simulink model "VehCtrlMdel240926_2018b_amkspdlimit"  (R2019b)
settings: Solver=FixedStepDiscrete  StartTime=0.0  StopTime=20  FixedStep=0.0005  RelTol=1e-3  EnableMultiTasking=on
values from neighbouring files (symbols this model uses):
  Ax_OffSet = 0.0    [VehCtrlMdelDictionary.sldd]
  Ay_OffSet = 0.0    [VehCtrlMdelDictionary.sldd]
  Caf = 460.0    [VehCtrlMdelDictionary.sldd]
  Car = 440.0    [VehCtrlMdelDictionary.sldd]
  dwf = 1.2    [VehCtrlMdelDictionary.sldd]
  dwr = 1.2    [VehCtrlMdelDictionary.sldd]
  h = 0.29    [VehCtrlMdelDictionary.sldd]
  i1 = 11.42    [VehCtrlMdelDictionary.sldd]
  i2 = 3.727    [VehCtrlMdelDictionary.sldd]
  Iz = 105.0    [VehCtrlMdelDictionary.sldd]
  Kc = 1.0    [VehCtrlMdelDictionary.sldd]
  Ki = 1.0    [VehCtrlMdelDictionary.sldd]
  Kp = 2.0    [VehCtrlMdelDictionary.sldd]
  Ldwf = 1.2    [VehCtrlMdelDictionary.sldd]
  Ldwr = 1.16    [VehCtrlMdelDictionary.sldd]
  lf = 0.761    [VehCtrlMdelDictionary.sldd]
  lr = 0.831    [VehCtrlMdelDictionary.sldd]
  m = 340.0    [VehCtrlMdelDictionary.sldd]
  Offset_Angle = 0.0    [VehCtrlMdelDictionary.sldd]
  Qa = 0.1    [VehCtrlMdelDictionary.sldd]
  Ra = 2.0    [VehCtrlMdelDictionary.sldd]
  Rt = 0.2    [VehCtrlMdelDictionary.sldd]
  thr1 = 2.0    [VehCtrlMdelDictionary.sldd]
  thr2 = 0.5    [VehCtrlMdelDictionary.sldd]
  thr3 = 0.8    [VehCtrlMdelDictionary.sldd]
  thr4 = 0.5    [VehCtrlMdelDictionary.sldd]
  thr5 = -0.5    [VehCtrlMdelDictionary.sldd]
  TrqRquRate = 0.1    [VehCtrlMdelDictionary.sldd]
  YawRate_OffSet = 0.0    [VehCtrlMdelDictionary.sldd]
undefined symbols (not defined in the file or in its folder): DiscIntNeverNeededParam, I_AN06_5V, I_AN07_5V, I_AN08_5V, I_AN09_5V, I_SW01_L, I_SW03_L, I_SW04_L, O_SW01_LS0A4, O_SW12_HS1A, O_SW13_HS1A, O_SW14_HS1A, O_SW15_HS1A, PWM3
libraries: simulink x152, ec5744lib x129, canmsglib x18
(part 5 of 6)

== system VehCtrlMdel240926_2018b_amkspdlimit/Input_Processing/Subsystem/WhlSlpageJudgment/速差判断 ==
  note: 输出“1”代表判定有效
  <VxFL_mps> : Inport
  <VxFR_mps> : Inport  Port=2
  <VxRL_mps> : Inport  Port=3
  <VxRR_mps> : Inport  Port=4
  VehSpd_mps : Inport  Port=5
  In6 : Inport  Port=6
  AND{,1..3} (4 alike) : Logic  AllPortsSameDT=off  OutDataTypeStr=boolean
  Abs{,1..3} (4 alike) : Abs
  Add{,1..3} (4 alike) : Sum  Inputs=+-
  Bus Selector1 : BusSelector  OutputSignals=WhlSpdii_mps.WhlSpdRL_Valid,WhlSpdii_mps.WhlSpdRR_Valid,WhlSpdii_mps.WhlSpdFR_Valid,WhlSpdii_mps.WhlSpdFL_Valid
  Compare To Constant{,1..3} (4 alike) : simulink/Logic and Bit Operations/Compare To Constant  relop=<=  const=thr1  OutDataTypeStr=boolean
  y : Outport
  y1 : Outport  Port=2
  y2 : Outport  Port=3
  y3 : Outport  Port=4
  wires:
  Add2/1 -> Abs2/1
  Abs1/1 -> Compare To Constant1/1
  <VxRR_mps>/1 -> Add3/1
  Add3/1 -> Abs3/1
  Add/1 -> Abs/1
  [VehSpd_mps] -> Add1/2
  <VxRL_mps>/1 -> Add2/1
  <VxFR_mps>/1 -> Add1/1
  Compare To Constant1/1 -> AND2/1
  Compare To Constant3/1 -> AND1/1
  Abs3/1 -> Compare To Constant3/1
  [VehSpd_mps] -> Add/2
  [VehSpd_mps] -> Add2/2
  [VehSpd_mps] -> Add3/2
  Abs/1 -> Compare To Constant/1
  Add1/1 -> Abs1/1
  Abs2/1 -> Compare To Constant2/1
  <VxFL_mps>/1 -> Add/1
  Compare To Constant2/1 -> AND/1
  Compare To Constant/1 -> AND3/1
  VehSpd_mps/1 -> [VehSpd_mps]
  In6/1 -> Bus Selector1/1
  Bus Selector1/1 -> AND/2  "<WhlSpdRL_Valid>"
  Bus Selector1/2 -> AND1/2  "<WhlSpdRR_Valid>"
  Bus Selector1/3 -> AND2/2  "<WhlSpdFR_Valid>"
  Bus Selector1/4 -> AND3/2  "<WhlSpdFL_Valid>"
  AND3/1 -> y/1
  AND2/1 -> y1/1
  AND1/1 -> y3/1
  AND/1 -> y2/1

== system VehCtrlMdel240926_2018b_amkspdlimit/Input_Processing/Subsystem/WhlSpdSelect/Filter ==
  In : Inport
  Add : Sum
  Constant : Constant  Value=single(0)
  Constant1 : Constant  Value=single(100)
  Constant2 : Constant  Value=single(15)
  Constant3 : Constant  Value=single(-15)
  Gain : Gain  Gain=0
  Gain1 : Gain
  Rate Limiter Dynamic : simulink/Discontinuities/Rate Limiter Dynamic
      settings: SourceProductName=Simulink
  Saturation Dynamic : simulink/Discontinuities/Saturation Dynamic  OutMin=[]  OutMax=[]  OutDataTypeStr=Inherit: Same as second input  OutDataType=fixdt(1, 16)  OutScaling=2^-10  DoSatur=off
  Unit Delay : UnitDelay  SampleTime=-1  HasFrameUpgradeWarning=on
  VehVxEst_mps : Outport
  wires:
  In/1 -> Saturation Dynamic/2
  Saturation Dynamic/1 -> Rate Limiter Dynamic/2
  Constant1/1 -> Saturation Dynamic/1
  Constant/1 -> Saturation Dynamic/3
  Unit Delay/1 -> Gain/1
  Gain/1 -> Add/1
  Gain1/1 -> Add/2
  Rate Limiter Dynamic/1 -> Gain1/1, Unit Delay/1
  Add/1 -> VehVxEst_mps/1
  Constant2/1 -> Rate Limiter Dynamic/1
  Constant3/1 -> Rate Limiter Dynamic/3

== system VehCtrlMdel240926_2018b_amkspdlimit/Input_Processing/Subsystem/WhlSpdSelect/Subsystem ==
  <VxFL_mps> : Inport
  <VxFR_mps> : Inport  Port=2
  <VxRL_mps> : Inport  Port=3
  <VxRR_mps> : Inport  Port=4
  Add3 : Sum  Inputs=++++
  Add4 : Sum  Inputs=+--
  Gain1 : Gain  Gain=1/2
  Min3 : MinMax  Function=max  Inputs=4
  Min4 : MinMax  Inputs=4
  Subsystem : Subsystem  Commented=on
  MiddleWhlSpd_mps : Outport
  wires:
  Add4/1 -> Gain1/1
  Add3/1 -> Add4/1
  Min3/1 -> Add4/3
  <VxRR_mps>/1 -> Min3/4, Add3/1, Min4/4
  <VxRL_mps>/1 -> Min3/3, Min4/3, Add3/2
  <VxFR_mps>/1 -> Min4/2, Min3/2, Add3/3
  Min4/1 -> Add4/2
  <VxFL_mps>/1 -> Add3/4, Min4/1, Min3/1
  Gain1/1 -> MiddleWhlSpd_mps/1  "MaxWhlSpd_mps"

== system VehCtrlMdel240926_2018b_amkspdlimit/Input/AMKMCU_Receive/FLAMKMCU/AMKMCU_state/MCU_state ==
  ID : Inport
  Msg : Inport  Port=2
  Enable : EnablePort
  Bus Creator : BusCreator  Inputs=12
  CAN Unpack : canmsglib/CAN Unpack  CANdbFile=d:\Users\YJR\Desktop\低压组\amk电机\DRe20_dbc_v1.16\DRe20_dbc_v1.16_CAN2.dbc  MsgList=MCFL_ActualValue1  MsgName=MCFL_ActualValue1  MsgIDType=Standard (11-bit identifier)  MsgIdentifier=640  MsgLength=8  SignalInfo={'MCFL_ActualTorque','32','16','LE','signed','Standard','0','0.0098','0','-Inf','Inf';'MCFL_ActualVelocity','48','16','LE','signed','Standard','0','1','0','-Inf','Inf';'MCFL_DCVoltage','16','16','LE','unsigned','Standard','0','1','0','-Inf','Inf';'MCFL_bDCOn','12','1','LE','unsigned','Standard','0','1','0','0','1';'MCFL_bDerating','15','1','LE','unsigned','Standard','0','1','0','0','1';'MCFL_bError','9','1','LE','unsigned','Standard','0','1','0','0','1';'MCFL_bInverterOn','14','1','LE','unsigned','Standard','0','1','0','0','1';'MCFL_bQuitDCOn','11','1','LE','unsigned','Standard','0','1','0','0','1';'MCFL_bQuitInverterOn','13','1','LE','unsigned','Standard','0','1','0','0','1';'MCFL_bReserve','0','8','LE','unsigned','Standard','0','1','0','0','255';'MCFL_bSystemReady','8','1','LE','unsigned','Standard','0','1','0','0','1';'MCFL_bWarn','10','1','LE','unsigned','Standard','0','1','0','0','1'}  IDPort=off  TimestampPort=off  ErrorPort=off  RemotePort=off  LengthPort=off  StatusPort=off  ApplyMinMax=off
      settings: SourceProductName=Simulink Real-Time  SourceProductBaseCode=XP  DataFormat=CANdb specified signals
  CANUnPackMessage4 : ec5744lib/RapidECU_U3/04CANCommunication/CANUnPackMessage  datalength=8  canmessagetype=Standard(11-bit ID)  sampletime=-1
      settings: SourceProductName=ECUCoder for MPC5744
  Gain : Gain  Gain=-1
  MeaModule1 : ec5744lib/RapidECU_U3/07Calibration/MeaModule  signal=MCFL_ActualVelocity
      settings: SourceProductName=ECUCoder for MPC5744
  MeaModule2 : ec5744lib/RapidECU_U3/07Calibration/MeaModule  signal=MCFL_DCVoltage
      settings: SourceProductName=ECUCoder for MPC5744
  MeaModule3 : ec5744lib/RapidECU_U3/07Calibration/MeaModule  signal=MCFL_bDCOn
      settings: SourceProductName=ECUCoder for MPC5744
  MeaModule4 : ec5744lib/RapidECU_U3/07Calibration/MeaModule  signal=MCFL_bError
      settings: SourceProductName=ECUCoder for MPC5744
  MeaModule5 : ec5744lib/RapidECU_U3/07Calibration/MeaModule  signal=MCFL_bInverterOn
      settings: SourceProductName=ECUCoder for MPC5744
  MeaModule6 : ec5744lib/RapidECU_U3/07Calibration/MeaModule  signal=MCFL_bQuitDCOn
      settings: SourceProductName=ECUCoder for MPC5744
  MeaModule7 : ec5744lib/RapidECU_U3/07Calibration/MeaModule  signal=MCFL_bQuitInverterOn
      settings: SourceProductName=ECUCoder for MPC5744
  MeaModule8 : ec5744lib/RapidECU_U3/07Calibration/MeaModule  signal=MCFL_bSystemReady
      settings: SourceProductName=ECUCoder for MPC5744
  MeaModule9 : ec5744lib/RapidECU_U3/07Calibration/MeaModule  signal=MCFL_ActualTorque
      settings: SourceProductName=ECUCoder for MPC5744
  FLAMKMCUtoVCU1 : Outport  VectorParamsAs1DForOutWhenUnconnected=off
  wires:
  Msg/1 -> CANUnPackMessage4/2
  ID/1 -> CANUnPackMessage4/1
  CANUnPackMessage4/1 -> CAN Unpack/1
  CAN Unpack/1 -> MeaModule9/1  "MCFL_ActualTorque"
  CAN Unpack/2 -> Gain/1  "MCFL_ActualVelocity"
  CAN Unpack/3 -> MeaModule2/1  "MCFL_DCVoltage"
  CAN Unpack/4 -> MeaModule3/1  "MCFL_bDCOn"
  CAN Unpack/5 -> Bus Creator/5  "MCFL_bDerating"
  CAN Unpack/6 -> MeaModule4/1  "MCFL_bError"
  CAN Unpack/7 -> MeaModule5/1  "MCFL_bInverterOn"
  CAN Unpack/8 -> MeaModule6/1  "MCFL_bQuitDCOn"
  CAN Unpack/9 -> MeaModule7/1  "MCFL_bQuitInverterOn"
  CAN Unpack/10 -> Bus Creator/10  "MCFL_bReserve"
  CAN Unpack/11 -> MeaModule8/1  "MCFL_bSystemReady"
  CAN Unpack/12 -> Bus Creator/12  "MCFL_bWarn"
  Bus Creator/1 -> FLAMKMCUtoVCU1/1  "FLAMKMCUtoVCU1"
  MeaModule1/1 -> Bus Creator/2
  MeaModule2/1 -> Bus Creator/3
  MeaModule3/1 -> Bus Creator/4
  MeaModule4/1 -> Bus Creator/6
  MeaModule5/1 -> Bus Creator/7
  MeaModule6/1 -> Bus Creator/8
  MeaModule7/1 -> Bus Creator/9
  MeaModule8/1 -> Bus Creator/11
  Gain/1 -> MeaModule1/1
  MeaModule9/1 -> Bus Creator/1  "MCFL_ActualTorque"

== system VehCtrlMdel240926_2018b_amkspdlimit/Input/AMKMCU_Receive/FLAMKMCU/AMKMCU_state1/MCU_state ==
  ID : Inport
  Msg : Inport  Port=2
  Enable : EnablePort
  CAN Unpack : canmsglib/CAN Unpack  CANdbFile=d:\Users\YJR\Desktop\低压组\amk电机\DRe20_dbc_v1.16\DRe20_dbc_v1.16_CAN2.dbc  MsgList=MCFL_ActualValue2  MsgName=MCFL_ActualValue2  MsgIDType=Standard (11-bit identifier)  MsgIdentifier=642  MsgLength=8  SignalInfo={'MCFL_DiagnosticNum','0','32','LE','unsigned','Standard','0','1','0','-Inf','Inf';'MCFL_ErrorInfo','32','32','LE','unsigned','Standard','0','1','0','-Inf','Inf'}  IDPort=off  TimestampPort=off  ErrorPort=off  RemotePort=off  LengthPort=off  StatusPort=off  ApplyMinMax=off
      settings: SourceProductName=Simulink Real-Time  SourceProductBaseCode=XP  DataFormat=CANdb specified signals
  CANUnPackMessage4 : ec5744lib/RapidECU_U3/04CANCommunication/CANUnPackMessage  datalength=8  canmessagetype=Standard(11-bit ID)  sampletime=-1
      settings: SourceProductName=ECUCoder for MPC5744
  MeaModule1 : ec5744lib/RapidECU_U3/07Calibration/MeaModule  signal=MCFL_ErrorInfo
      settings: SourceProductName=ECUCoder for MPC5744
  MCFL_DiagnosticNum : Outport  VectorParamsAs1DForOutWhenUnconnected=off
  MCFL_ErrorInfo : Outport  Port=2  VectorParamsAs1DForOutWhenUnconnected=off
  wires:
  CANUnPackMessage4/1 -> CAN Unpack/1
  ID/1 -> CANUnPackMessage4/1
  Msg/1 -> CANUnPackMessage4/2
  CAN Unpack/1 -> MCFL_DiagnosticNum/1  "MCFL_DiagnosticNum"
  CAN Unpack/2 -> MeaModule1/1  "MCFL_ErrorInfo"
  MeaModule1/1 -> MCFL_ErrorInfo/1

== system VehCtrlMdel240926_2018b_amkspdlimit/Input/AMKMCU_Receive/FLAMKMCU/AMKMCU_state2/MCU_state ==
  ID : Inport
  Msg : Inport  Port=2
  Enable : EnablePort
  CAN Unpack : canmsglib/CAN Unpack  CANdbFile=d:\Users\YJR\Desktop\低压组\amk电机\DRe20_dbc_v1.16\DRe20_dbc_v1.16_CAN2.dbc  MsgList=MCFL_ActualValue3  MsgName=MCFL_ActualValue3  MsgIDType=Standard (11-bit identifier)  MsgIdentifier=644  MsgLength=6  SignalInfo={'MCFL_TempIGBT','32','16','LE','unsigned','Standard','0','0.1','0','-Inf','Inf';'MCFL_TempInverter','16','16','LE','unsigned','Standard','0','0.1','0','-Inf','Inf';'MCFL_TempMotor','0','16','LE','unsigned','Standard','0','0.1','0','-Inf','Inf'}  IDPort=off  TimestampPort=off  ErrorPort=off  RemotePort=off  LengthPort=off  StatusPort=off  ApplyMinMax=off
      settings: SourceProductName=Simulink Real-Time  SourceProductBaseCode=XP  DataFormat=CANdb specified signals
  CANUnPackMessage4 : ec5744lib/RapidECU_U3/04CANCommunication/CANUnPackMessage  datalength=6  canmessagetype=Standard(11-bit ID)  sampletime=-1
      settings: SourceProductName=ECUCoder for MPC5744
  MeaModule1 : ec5744lib/RapidECU_U3/07Calibration/MeaModule  signal=MCFL_TempIGBT
      settings: SourceProductName=ECUCoder for MPC5744
  MeaModule2 : ec5744lib/RapidECU_U3/07Calibration/MeaModule  signal=MCFL_TempInverter
      settings: SourceProductName=ECUCoder for MPC5744
  MeaModule3 : ec5744lib/RapidECU_U3/07Calibration/MeaModule  signal=MCFL_TempMotor
      settings: SourceProductName=ECUCoder for MPC5744
  MCFL_TempIGBT : Outport  VectorParamsAs1DForOutWhenUnconnected=off
  MCFL_TempInverter : Outport  Port=2  VectorParamsAs1DForOutWhenUnconnected=off
  MCFL_TempMotor : Outport  Port=3  VectorParamsAs1DForOutWhenUnconnected=off
  wires:
  Msg/1 -> CANUnPackMessage4/2
  ID/1 -> CANUnPackMessage4/1
  CANUnPackMessage4/1 -> CAN Unpack/1
  CAN Unpack/1 -> MeaModule1/1  "MCFL_TempIGBT"
  CAN Unpack/2 -> MeaModule2/1  "MCFL_TempInverter"
  CAN Unpack/3 -> MeaModule3/1  "MCFL_TempMotor"
  MeaModule1/1 -> MCFL_TempIGBT/1
  MeaModule2/1 -> MCFL_TempInverter/1
  MeaModule3/1 -> MCFL_TempMotor/1

== system VehCtrlMdel240926_2018b_amkspdlimit/Input/AMKMCU_Receive/FRAMKMCU/AMKMCU_state/MCU_state ==
  ID : Inport
  Msg : Inport  Port=2
  Enable : EnablePort
  CAN Unpack : canmsglib/CAN Unpack  CANdbFile=d:\Users\YJR\Desktop\低压组\amk电机\DRe20_dbc_v1.16\DRe20_dbc_v1.16_CAN2.dbc  MsgList=MCFR_ActualValue1  MsgName=MCFR_ActualValue1  MsgIDType=Standard (11-bit identifier)  MsgIdentifier=641  MsgLength=8  SignalInfo={'MCFR_ActualTorque','32','16','LE','signed','Standard','0','0.0098','0','-Inf','Inf';'MCFR_ActualVelocity','48','16','LE','signed','Standard','0','1','0','-Inf','Inf';'MCFR_DCVoltage','16','16','LE','unsigned','Standard','0','1','0','-Inf','Inf';'MCFR_bDCOn','12','1','LE','unsigned','Standard','0','1','0','0','1';'MCFR_bDerating','15','1','LE','unsigned','Standard','0','1','0','0','1';'MCFR_bError','9','1','LE','unsigned','Standard','0','1','0','0','1';'MCFR_bInverterOn','14','1','LE','unsigned','Standard','0','1','0','0','1';'MCFR_bQuitDCOn','11','1','LE','unsigned','Standard','0','1','0','0','1';'MCFR_bQuitInverterOn','13','1','LE','unsigned','Standard','0','1','0','0','1';'MCFR_bReserve','0','8','LE','unsigned','Standard','0','1','0','0','255';'MCFR_bSystemReady','8','1','LE','unsigned','Standard','0','1','0','0','1';'MCFR_bWarn','10','1','LE','unsigned','Standard','0','1','0','0','1'}  IDPort=off  TimestampPort=off  ErrorPort=off  RemotePort=off  LengthPort=off  StatusPort=off  ApplyMinMax=off
      settings: SourceProductName=Simulink Real-Time  SourceProductBaseCode=XP  DataFormat=CANdb specified signals
  CANUnPackMessage4 : ec5744lib/RapidECU_U3/04CANCommunication/CANUnPackMessage  datalength=8  canmessagetype=Standard(11-bit ID)  sampletime=-1
      settings: SourceProductName=ECUCoder for MPC5744
  MeaModule1 : ec5744lib/RapidECU_U3/07Calibration/MeaModule  signal=MCFR_ActualVelocity
      settings: SourceProductName=ECUCoder for MPC5744
  MeaModule2 : ec5744lib/RapidECU_U3/07Calibration/MeaModule  signal=MCFR_DCVoltage
      settings: SourceProductName=ECUCoder for MPC5744
  MeaModule3 : ec5744lib/RapidECU_U3/07Calibration/MeaModule  signal=MCFR_bDCOn
      settings: SourceProductName=ECUCoder for MPC5744
  MeaModule4 : ec5744lib/RapidECU_U3/07Calibration/MeaModule  signal=MCFR_bError
      settings: SourceProductName=ECUCoder for MPC5744
  MeaModule5 : ec5744lib/RapidECU_U3/07Calibration/MeaModule  signal=MCFR_bInverterOn
      settings: SourceProductName=ECUCoder for MPC5744
  MeaModule6 : ec5744lib/RapidECU_U3/07Calibration/MeaModule  signal=MCFR_bQuitInverterOn
      settings: SourceProductName=ECUCoder for MPC5744
  MeaModule7 : ec5744lib/RapidECU_U3/07Calibration/MeaModule  signal=MCFR_bSystemReady
      settings: SourceProductName=ECUCoder for MPC5744
  MeaModule8 : ec5744lib/RapidECU_U3/07Calibration/MeaModule  signal=MCFR_ActualTorque
      settings: SourceProductName=ECUCoder for MPC5744
  MCFR_ActualTorque : Outport  VectorParamsAs1DForOutWhenUnconnected=off
  MCFR_ActualVelocity : Outport  Port=2  VectorParamsAs1DForOutWhenUnconnected=off
  MCFR_DCVoltage : Outport  Port=3  VectorParamsAs1DForOutWhenUnconnected=off
  MCFR_bDCOn : Outport  Port=4  VectorParamsAs1DForOutWhenUnconnected=off
  MCFR_bDerating : Outport  Port=5  VectorParamsAs1DForOutWhenUnconnected=off
  MCFR_bError : Outport  Port=6  VectorParamsAs1DForOutWhenUnconnected=off
  MCFR_bInverterOn : Outport  Port=7  VectorParamsAs1DForOutWhenUnconnected=off
  MCFR_bQuitDCOn : Outport  Port=8  VectorParamsAs1DForOutWhenUnconnected=off
  MCFR_bQuitInverterOn : Outport  Port=9  VectorParamsAs1DForOutWhenUnconnected=off
  MCFR_bReserve : Outport  Port=10  VectorParamsAs1DForOutWhenUnconnected=off
  MCFR_bSystemReady : Outport  Port=11  VectorParamsAs1DForOutWhenUnconnected=off
  MCFR_bWarn : Outport  Port=12  VectorParamsAs1DForOutWhenUnconnected=off
  wires:
  CANUnPackMessage4/1 -> CAN Unpack/1
  ID/1 -> CANUnPackMessage4/1
  Msg/1 -> CANUnPackMessage4/2
  CAN Unpack/1 -> MeaModule8/1  "MCFR_ActualTorque"
  CAN Unpack/2 -> MeaModule1/1  "MCFR_ActualVelocity"
  CAN Unpack/4 -> MeaModule3/1  "MCFR_bDCOn"
  CAN Unpack/3 -> MeaModule2/1  "MCFR_DCVoltage"
  CAN Unpack/7 -> MeaModule5/1  "MCFR_bInverterOn"
  CAN Unpack/5 -> MCFR_bDerating/1  "MCFR_bDerating"
  CAN Unpack/6 -> MeaModule4/1  "MCFR_bError"
  CAN Unpack/8 -> MCFR_bQuitDCOn/1  "MCFR_bQuitDCOn"
  CAN Unpack/9 -> MeaModule6/1  "MCFR_bQuitInverterOn"
  CAN Unpack/10 -> MCFR_bReserve/1  "MCFR_bReserve"
  CAN Unpack/11 -> MeaModule7/1  "MCFR_bSystemReady"
  CAN Unpack/12 -> MCFR_bWarn/1  "MCFR_bWarn"
  MeaModule1/1 -> MCFR_ActualVelocity/1
  MeaModule2/1 -> MCFR_DCVoltage/1
  MeaModule3/1 -> MCFR_bDCOn/1
  MeaModule4/1 -> MCFR_bError/1
  MeaModule5/1 -> MCFR_bInverterOn/1
  MeaModule6/1 -> MCFR_bQuitInverterOn/1
  MeaModule7/1 -> MCFR_bSystemReady/1
  MeaModule8/1 -> MCFR_ActualTorque/1  "MCFR_ActualTorque"

== system VehCtrlMdel240926_2018b_amkspdlimit/Input/AMKMCU_Receive/FRAMKMCU/AMKMCU_state1/MCU_state ==
  ID : Inport
  Msg : Inport  Port=2
  Enable : EnablePort
  CAN Unpack : canmsglib/CAN Unpack  CANdbFile=d:\Users\YJR\Desktop\低压组\amk电机\DRe20_dbc_v1.16\DRe20_dbc_v1.16_CAN2.dbc  MsgList=MCFR_ActualValue2  MsgName=MCFR_ActualValue2  MsgIDType=Standard (11-bit identifier)  MsgIdentifier=643  MsgLength=8  SignalInfo={'MCFR_DiagnosticNum','0','32','LE','unsigned','Standard','0','1','0','-Inf','Inf';'MCFR_ErrorInfo','32','32','LE','unsigned','Standard','0','1','0','-Inf','Inf'}  IDPort=off  TimestampPort=off  ErrorPort=off  RemotePort=off  LengthPort=off  StatusPort=off  ApplyMinMax=off
      settings: SourceProductName=Simulink Real-Time  SourceProductBaseCode=XP  DataFormat=CANdb specified signals
  CANUnPackMessage4 : ec5744lib/RapidECU_U3/04CANCommunication/CANUnPackMessage  datalength=8  canmessagetype=Standard(11-bit ID)  sampletime=-1
      settings: SourceProductName=ECUCoder for MPC5744
  MeaModule1 : ec5744lib/RapidECU_U3/07Calibration/MeaModule  signal=MCFR_ErrorInfo
      settings: SourceProductName=ECUCoder for MPC5744
  MCFR_DiagnosticNum : Outport  VectorParamsAs1DForOutWhenUnconnected=off
  MCFR_ErrorInfo : Outport  Port=2  VectorParamsAs1DForOutWhenUnconnected=off
  wires:
  Msg/1 -> CANUnPackMessage4/2
  ID/1 -> CANUnPackMessage4/1
  CANUnPackMessage4/1 -> CAN Unpack/1
  CAN Unpack/1 -> MCFR_DiagnosticNum/1  "MCFR_DiagnosticNum"
  CAN Unpack/2 -> MeaModule1/1  "MCFR_ErrorInfo"
  MeaModule1/1 -> MCFR_ErrorInfo/1

== system VehCtrlMdel240926_2018b_amkspdlimit/Input/AMKMCU_Receive/FRAMKMCU/AMKMCU_state2/MCU_state ==
  ID : Inport
  Msg : Inport  Port=2
  Enable : EnablePort
  CAN Unpack : canmsglib/CAN Unpack  CANdbFile=d:\Users\YJR\Desktop\低压组\amk电机\DRe20_dbc_v1.16\DRe20_dbc_v1.16_CAN2.dbc  MsgList=MCFR_ActualValue3  MsgName=MCFR_ActualValue3  MsgIDType=Standard (11-bit identifier)  MsgIdentifier=645  MsgLength=6  SignalInfo={'MCFR_TempIGBT','32','16','LE','unsigned','Standard','0','0.1','0','-Inf','Inf';'MCFR_TempInverter','16','16','LE','unsigned','Standard','0','0.1','0','-Inf','Inf';'MCFR_TempMotor','0','16','LE','unsigned','Standard','0','0.1','0','-Inf','Inf'}  IDPort=off  TimestampPort=off  ErrorPort=off  RemotePort=off  LengthPort=off  StatusPort=off  ApplyMinMax=off
      settings: SourceProductName=Simulink Real-Time  SourceProductBaseCode=XP  DataFormat=CANdb specified signals
  CANUnPackMessage4 : ec5744lib/RapidECU_U3/04CANCommunication/CANUnPackMessage  datalength=6  canmessagetype=Standard(11-bit ID)  sampletime=-1
      settings: SourceProductName=ECUCoder for MPC5744
  MeaModule1 : ec5744lib/RapidECU_U3/07Calibration/MeaModule  signal=MCFR_TempIGBT
      settings: SourceProductName=ECUCoder for MPC5744
  MeaModule2 : ec5744lib/RapidECU_U3/07Calibration/MeaModule  signal=MCFR_TempInverter
      settings: SourceProductName=ECUCoder for MPC5744
  MeaModule3 : ec5744lib/RapidECU_U3/07Calibration/MeaModule  signal=MCFR_TempMotor
      settings: SourceProductName=ECUCoder for MPC5744
  MCFR_TempIGBT : Outport  VectorParamsAs1DForOutWhenUnconnected=off
  MCFR_TempInverter : Outport  Port=2  VectorParamsAs1DForOutWhenUnconnected=off
  MCFR_TempMotor : Outport  Port=3  VectorParamsAs1DForOutWhenUnconnected=off
  wires:
  CANUnPackMessage4/1 -> CAN Unpack/1
  ID/1 -> CANUnPackMessage4/1
  Msg/1 -> CANUnPackMessage4/2
  CAN Unpack/1 -> MeaModule1/1  "MCFR_TempIGBT"
  CAN Unpack/2 -> MeaModule2/1  "MCFR_TempInverter"
  CAN Unpack/3 -> MeaModule3/1  "MCFR_TempMotor"
  MeaModule1/1 -> MCFR_TempIGBT/1
  MeaModule2/1 -> MCFR_TempInverter/1
  MeaModule3/1 -> MCFR_TempMotor/1

== system VehCtrlMdel240926_2018b_amkspdlimit/Input_Processing/Subsystem/WhlSlpageJudgment/加速度差判断/Filter ==
  In : Inport
  Add : Sum
  Constant : Constant  Value=single(-100)
  Constant1 : Constant  Value=single(100)
  Constant2 : Constant  Value=single(100)
  Constant3 : Constant  Value=single(-100)
  Gain : Gain  Gain=0.3
  Gain1 : Gain  Gain=0.7
  Rate Limiter Dynamic : simulink/Discontinuities/Rate Limiter Dynamic
      settings: SourceProductName=Simulink
  Saturation Dynamic : simulink/Discontinuities/Saturation Dynamic  OutMin=[]  OutMax=[]  OutDataTypeStr=Inherit: Same as second input  OutDataType=fixdt(1, 16)  OutScaling=2^-10  DoSatur=off
  Unit Delay : UnitDelay  SampleTime=-1  HasFrameUpgradeWarning=on
  Out : Outport
  wires:
  In/1 -> Saturation Dynamic/2
  Saturation Dynamic/1 -> Rate Limiter Dynamic/2
  Constant1/1 -> Saturation Dynamic/1
  Constant/1 -> Saturation Dynamic/3
  Constant2/1 -> Rate Limiter Dynamic/1
  Constant3/1 -> Rate Limiter Dynamic/3
  Unit Delay/1 -> Gain/1
  Gain/1 -> Add/1
  Add/1 -> Out/1
  Gain1/1 -> Add/2
  Rate Limiter Dynamic/1 -> Gain1/1, Unit Delay/1

== system VehCtrlMdel240926_2018b_amkspdlimit/Input_Processing/Subsystem/WhlSlpageJudgment/加速度差判断/Filter1 ==
  In : Inport
  Add : Sum
  Constant : Constant  Value=single(-100)
  Constant1 : Constant  Value=single(100)
  Constant2 : Constant  Value=single(100)
  Constant3 : Constant  Value=single(-100)
  Gain : Gain  Gain=0.3
  Gain1 : Gain  Gain=0.7
  Rate Limiter Dynamic : simulink/Discontinuities/Rate Limiter Dynamic
      settings: SourceProductName=Simulink
  Saturation Dynamic : simulink/Discontinuities/Saturation Dynamic  OutMin=[]  OutMax=[]  OutDataTypeStr=Inherit: Same as second input  OutDataType=fixdt(1, 16)  OutScaling=2^-10  DoSatur=off
  Unit Delay : UnitDelay  SampleTime=-1  HasFrameUpgradeWarning=on
  Out : Outport
  wires:
  Rate Limiter Dynamic/1 -> Unit Delay/1, Gain1/1
  Gain1/1 -> Add/2
  Add/1 -> Out/1
  Gain/1 -> Add/1
  Unit Delay/1 -> Gain/1
  Constant3/1 -> Rate Limiter Dynamic/3
  Constant2/1 -> Rate Limiter Dynamic/1
  Constant/1 -> Saturation Dynamic/3
  Constant1/1 -> Saturation Dynamic/1
  Saturation Dynamic/1 -> Rate Limiter Dynamic/2
  In/1 -> Saturation Dynamic/2

== system VehCtrlMdel240926_2018b_amkspdlimit/Input_Processing/Subsystem/WhlSlpageJudgment/加速度差判断/Filter2 ==
  In : Inport
  Add : Sum
  Constant : Constant  Value=single(-100)
  Constant1 : Constant  Value=single(100)
  Constant2 : Constant  Value=single(100)
  Constant3 : Constant  Value=single(-100)
  Gain : Gain  Gain=0.3
  Gain1 : Gain  Gain=0.7
  Rate Limiter Dynamic : simulink/Discontinuities/Rate Limiter Dynamic
      settings: SourceProductName=Simulink
  Saturation Dynamic : simulink/Discontinuities/Saturation Dynamic  OutMin=[]  OutMax=[]  OutDataTypeStr=Inherit: Same as second input  OutDataType=fixdt(1, 16)  OutScaling=2^-10  DoSatur=off
  Unit Delay : UnitDelay  SampleTime=-1  HasFrameUpgradeWarning=on
  Out : Outport
  wires:
  In/1 -> Saturation Dynamic/2
  Saturation Dynamic/1 -> Rate Limiter Dynamic/2
  Constant1/1 -> Saturation Dynamic/1
  Constant/1 -> Saturation Dynamic/3
  Constant2/1 -> Rate Limiter Dynamic/1
  Constant3/1 -> Rate Limiter Dynamic/3
  Unit Delay/1 -> Gain/1
  Gain/1 -> Add/1
  Add/1 -> Out/1
  Gain1/1 -> Add/2
  Rate Limiter Dynamic/1 -> Gain1/1, Unit Delay/1

== system VehCtrlMdel240926_2018b_amkspdlimit/Input_Processing/Subsystem/WhlSlpageJudgment/加速度差判断/Filter3 ==
  In : Inport
  Add : Sum
  Constant : Constant  Value=single(-100)
  Constant1 : Constant  Value=single(100)
  Constant2 : Constant  Value=single(100)
  Constant3 : Constant  Value=single(-100)
  Gain : Gain  Gain=0.3
  Gain1 : Gain  Gain=0.7
  Rate Limiter Dynamic : simulink/Discontinuities/Rate Limiter Dynamic
      settings: SourceProductName=Simulink
  Saturation Dynamic : simulink/Discontinuities/Saturation Dynamic  OutMin=[]  OutMax=[]  OutDataTypeStr=Inherit: Same as second input  OutDataType=fixdt(1, 16)  OutScaling=2^-10  DoSatur=off
  Unit Delay : UnitDelay  SampleTime=-1  HasFrameUpgradeWarning=on
  Out : Outport
  wires:
  Rate Limiter Dynamic/1 -> Unit Delay/1, Gain1/1
  Gain1/1 -> Add/2
  Add/1 -> Out/1
  Gain/1 -> Add/1
  Unit Delay/1 -> Gain/1
  Constant3/1 -> Rate Limiter Dynamic/3
  Constant2/1 -> Rate Limiter Dynamic/1
  Constant/1 -> Saturation Dynamic/3
  Constant1/1 -> Saturation Dynamic/1
  Saturation Dynamic/1 -> Rate Limiter Dynamic/2
  In/1 -> Saturation Dynamic/2

== system VehCtrlMdel240926_2018b_amkspdlimit/Input_Processing/Subsystem/WhlSlpageJudgment/加速度差的微分的判断/Filter ==
  In : Inport
  Add : Sum
  Constant : Constant  Value=single(-100)
  Constant1 : Constant  Value=single(100)
  Constant2 : Constant  Value=single(20)
  Constant3 : Constant  Value=single(-20)
  Gain : Gain  Gain=0.5
  Gain1 : Gain  Gain=0.5
  Rate Limiter Dynamic : simulink/Discontinuities/Rate Limiter Dynamic
      settings: SourceProductName=Simulink
  Saturation Dynamic : simulink/Discontinuities/Saturation Dynamic  OutMin=[]  OutMax=[]  OutDataTypeStr=Inherit: Same as second input  OutDataType=fixdt(1, 16)  OutScaling=2^-10  DoSatur=off
  Unit Delay : UnitDelay  SampleTime=-1  HasFrameUpgradeWarning=on
  Out : Outport
  wires:
  In/1 -> Saturation Dynamic/2
  Saturation Dynamic/1 -> Rate Limiter Dynamic/2
  Constant1/1 -> Saturation Dynamic/1
  Constant/1 -> Saturation Dynamic/3
  Constant2/1 -> Rate Limiter Dynamic/1
  Constant3/1 -> Rate Limiter Dynamic/3
  Unit Delay/1 -> Gain/1
  Gain/1 -> Add/1
  Add/1 -> Out/1
  Gain1/1 -> Add/2
  Rate Limiter Dynamic/1 -> Gain1/1, Unit Delay/1

== system VehCtrlMdel240926_2018b_amkspdlimit/Input_Processing/Subsystem/WhlSlpageJudgment/加速度差的微分的判断/Filter1 ==
  In : Inport
  Add : Sum
  Constant : Constant  Value=single(-100)
  Constant1 : Constant  Value=single(100)
  Constant2 : Constant  Value=single(20)
  Constant3 : Constant  Value=single(-20)
  Gain : Gain  Gain=0.5
  Gain1 : Gain  Gain=0.5
  Rate Limiter Dynamic : simulink/Discontinuities/Rate Limiter Dynamic
      settings: SourceProductName=Simulink
  Saturation Dynamic : simulink/Discontinuities/Saturation Dynamic  OutMin=[]  OutMax=[]  OutDataTypeStr=Inherit: Same as second input  OutDataType=fixdt(1, 16)  OutScaling=2^-10  DoSatur=off
  Unit Delay : UnitDelay  SampleTime=-1  HasFrameUpgradeWarning=on
  Out : Outport
  wires:
  Rate Limiter Dynamic/1 -> Unit Delay/1, Gain1/1
  Gain1/1 -> Add/2
  Add/1 -> Out/1
  Gain/1 -> Add/1
  Unit Delay/1 -> Gain/1
  Constant3/1 -> Rate Limiter Dynamic/3
  Constant2/1 -> Rate Limiter Dynamic/1
  Constant/1 -> Saturation Dynamic/3
  Constant1/1 -> Saturation Dynamic/1
  Saturation Dynamic/1 -> Rate Limiter Dynamic/2
  In/1 -> Saturation Dynamic/2

== system VehCtrlMdel240926_2018b_amkspdlimit/Input_Processing/Subsystem/WhlSlpageJudgment/加速度差的微分的判断/Filter2 ==
  In : Inport
  Add : Sum
  Constant : Constant  Value=single(-100)
  Constant1 : Constant  Value=single(100)
  Constant2 : Constant  Value=single(20)
  Constant3 : Constant  Value=single(-20)
  Gain : Gain  Gain=0.5
  Gain1 : Gain  Gain=0.5
  Rate Limiter Dynamic : simulink/Discontinuities/Rate Limiter Dynamic
      settings: SourceProductName=Simulink
  Saturation Dynamic : simulink/Discontinuities/Saturation Dynamic  OutMin=[]  OutMax=[]  OutDataTypeStr=Inherit: Same as second input  OutDataType=fixdt(1, 16)  OutScaling=2^-10  DoSatur=off
  Unit Delay : UnitDelay  SampleTime=-1  HasFrameUpgradeWarning=on
  Out : Outport
  wires:
  In/1 -> Saturation Dynamic/2
  Saturation Dynamic/1 -> Rate Limiter Dynamic/2
  Constant1/1 -> Saturation Dynamic/1
  Constant/1 -> Saturation Dynamic/3
  Constant2/1 -> Rate Limiter Dynamic/1
  Constant3/1 -> Rate Limiter Dynamic/3
  Unit Delay/1 -> Gain/1
  Gain/1 -> Add/1
  Add/1 -> Out/1
  Gain1/1 -> Add/2
  Rate Limiter Dynamic/1 -> Gain1/1, Unit Delay/1

== system VehCtrlMdel240926_2018b_amkspdlimit/Input_Processing/Subsystem/WhlSlpageJudgment/加速度差的微分的判断/Filter3 ==
  In : Inport
  Add : Sum
  Constant : Constant  Value=single(-100)
  Constant1 : Constant  Value=single(100)
  Constant2 : Constant  Value=single(20)
  Constant3 : Constant  Value=single(-20)
  Gain : Gain  Gain=0.5
  Gain1 : Gain  Gain=0.5
  Rate Limiter Dynamic : simulink/Discontinuities/Rate Limiter Dynamic
      settings: SourceProductName=Simulink
  Saturation Dynamic : simulink/Discontinuities/Saturation Dynamic  OutMin=[]  OutMax=[]  OutDataTypeStr=Inherit: Same as second input  OutDataType=fixdt(1, 16)  OutScaling=2^-10  DoSatur=off
  Unit Delay : UnitDelay  SampleTime=-1  HasFrameUpgradeWarning=on
  Out : Outport
  wires:
  Rate Limiter Dynamic/1 -> Unit Delay/1, Gain1/1
  Gain1/1 -> Add/2
  Add/1 -> Out/1
  Gain/1 -> Add/1
  Unit Delay/1 -> Gain/1
  Constant3/1 -> Rate Limiter Dynamic/3
  Constant2/1 -> Rate Limiter Dynamic/1
  Constant/1 -> Saturation Dynamic/3
  Constant1/1 -> Saturation Dynamic/1
  Saturation Dynamic/1 -> Rate Limiter Dynamic/2
  In/1 -> Saturation Dynamic/2

== system VehCtrlMdel240926_2018b_amkspdlimit/Input_Processing/Subsystem/WhlSpdSelect/Subsystem/Subsystem ==
  note: 可在去掉最大最小值里再取最大、最小
  In1 : Inport
  In2 : Inport  Port=2
  In3 : Inport  Port=3
  In4 : Inport  Port=4
  Add : Sum  Commented=on  Inputs=++++
  Add1 : Sum  Commented=on  Inputs=+--
  Add2 : Sum  Commented=on  Inputs=-+
  Compare To Constant1 : simulink/Logic and Bit Operations/Compare To Constant  Commented=on  relop=>  const=0.2  OutDataTypeStr=boolean
  Compare To Constant2 : simulink/Logic and Bit Operations/Compare To Constant  Commented=on  relop=<  const=-0.2  OutDataTypeStr=boolean
  Divide1 : Product  Commented=on  Inputs=*/
  Gain : Gain  Commented=on  Gain=1/2
  Max : MinMax  Commented=on  Function=max  Inputs=3
  Max1 : MinMax  Commented=on  Function=max  Inputs=3
  Max2 : MinMax  Commented=on  Inputs=2
  Max3 : MinMax  Commented=on  Inputs=3
  Max4 : MinMax  Commented=on  Inputs=3
  Max5 : MinMax  Commented=on  Function=max  Inputs=2
  Min1 : MinMax  Commented=on  Function=max  Inputs=4
  Min2 : MinMax  Commented=on  Inputs=4
  NOT : Logic  Commented=on  Operator=NOT  AllPortsSameDT=off  OutDataTypeStr=boolean
  Switch : Switch  Commented=on  Criteria=u2 ~= 0
  Switch1 : Switch  Commented=on  Criteria=u2 ~= 0
  Unit Delay1 : UnitDelay  Commented=on  SampleTime=-1  HasFrameUpgradeWarning=on
  steptime1 : Constant  Commented=on  Value=single(0.01)
  Out1 : Outport
  wires:
  Gain/1 -> Switch/3, Unit Delay1/1, Add2/2  "MaxWhlSpd_mps"
  Add2/1 -> Divide1/1
  In1/1 -> Max/1, Max3/1, Add/4, Min1/1, Min2/1
  In4/1 -> Max1/3, Max4/3, Add/1, Min1/4, Min2/4
  In2/1 -> Max/2, Max3/2, Max1/1, Max4/1, Add/3, Min1/2, Min2/2
  In3/1 -> Max/3, Max3/3, Add/2, Min1/3, Min2/3, Max1/2, Max4/2
  Max5/1 -> Switch1/3
  Unit Delay1/1 -> Add2/1
  Max4/1 -> Max5/2
  Compare To Constant2/1 -> Switch/2
  Max3/1 -> Max5/1
  steptime1/1 -> Divide1/2
  Add/1 -> Add1/1
  Compare To Constant1/1 -> NOT/1
  Divide1/1 -> Compare To Constant1/1, Compare To Constant2/1
  Min2/1 -> Add1/2
  Switch1/1 -> Out1/1
  Add1/1 -> Gain/1
  NOT/1 -> Switch1/2
  Max2/1 -> Switch/1
  Max/1 -> Max2/1
  Max1/1 -> Max2/2
  Switch/1 -> Switch1/1
  Min1/1 -> Add1/3

== stateflow chart VehCtrlMdel240926_2018b_amkspdlimit/Drive_Ready/Subsystem/Chart2 ==
  state VehStat [parallel]
    settings: executionOrder=1
    state WaitForEngine
      en:
      send(AMKCANOFF,AMKCANenable);
      send(AMKDCOFF,AMKDCon);
      send(MCDCEnableOFF,MCDCEnable);
      send(InverterFLOFF,MCFL_InverterOn);
      send(InverterFROFF,MCFR_InverterOn);
      send(TorqueOFF,MC_TorqueCUT);
      errorReset = 0;
    state Standby
    state Trans
    state Guard
    state InitStateBack
    state Ready
    state Init
      en:
      errorReset = 1;
    state MCUReadyFail
    WaitForEngine -> Standby : [aMCUReady&&bMCUReady&&cMCUReady]
    Standby -> Guard [order 2] : [KeyPressed&&Brk&&ACC_Release&&cMCUReady&&aMCUReady&&bMCUReady&&aQuitInverterOn&&bQuitInverterOn]
    Trans -> Ready : after(2.5,sec){send(EbeepOFF,BeeperStat)}
    Guard -> Trans [order 1] : after(0.25,sec){send(EbeepON,BeeperStat)}
    Guard -> Standby [order 2] : [~KeyPressed||~Brk||~ACC_Release]
    Standby -> WaitForEngine [order 1] : [~aMCUReady||~bMCUReady||~cMCUReady]
    Guard -> InitStateBack [order 3] : [~cMCUReady||~aMCUReady||~bMCUReady]
    Init -> WaitForEngine : [after(0.1,sec)]
    MCUReadyFail -> WaitForEngine
    InitStateBack -> WaitForEngine
    (default) -> Init
    Ready -> MCUReadyFail : [~cMCUReady||~aMCUReady||~bMCUReady]
  state BeeperStat [parallel]
    settings: executionOrder=2
    state OFF
    state ON
    (default) -> BeeperStat.OFF
    BeeperStat.OFF -> BeeperStat.ON : EbeepON
    BeeperStat.ON -> BeeperStat.OFF : EbeepOFF
  state AMKDCon [parallel]
    settings: executionOrder=3
    state OFF
    state ON
    (default) -> AMKDCon.OFF
    AMKDCon.OFF -> AMKDCon.ON : AMKDCON
    AMKDCon.ON -> AMKDCon.OFF : AMKDCOFF
  state MCDCEnable [parallel]
    settings: executionOrder=4
    state OFF
    state ON
    (default) -> MCDCEnable.OFF
    MCDCEnable.OFF -> MCDCEnable.ON : MCDCEnableON
    MCDCEnable.ON -> MCDCEnable.OFF : MCDCEnableOFF
  state MC_TorqueCUT [parallel]
    settings: executionOrder=5
    state OFF
    state ON
    (default) -> MC_TorqueCUT.OFF
    MC_TorqueCUT.OFF -> MC_TorqueCUT.ON : TorqueON
    MC_TorqueCUT.ON -> MC_TorqueCUT.OFF : TorqueOFF
  state AMKDCready [parallel]
    settings: executionOrder=6
    state start
    state AMKCAN
      en:
      send(AMKCANON,AMKCANenable);
    state MC_DCready
    state MCDCOncheck
    state DCOnCheckPass
    state SYSRDYCECK
    state AMKDCOnFinish
      en:
      send(TorqueON,MC_TorqueCUT);
    state MCFR_InverterOn_State
      en:
      send(InverterFRON,MCFR_InverterOn);
    state MCFL_InverterOn_State
      en:
      send(InverterFLON,MCFL_InverterOn);
    state MCDCEnableState
      en:
      send(MCDCEnableON,MCDCEnable);
    (default) -> start
    MC_DCready -> MCDCOncheck : after(0.5,sec){send(AMKDCON,AMKDCon)}
    MCDCOncheck -> DCOnCheckPass : after(1,sec)
    AMKCAN -> MC_DCready : [KeyPressed&&Brk&&ACC_Release]
    start -> AMKCAN : after(5,sec)
    DCOnCheckPass -> MCDCEnableState : after(1,sec)[MCFLDCOncheck&&MCFRDCOncheck]
    SYSRDYCECK -> AMKDCOnFinish : after(8,sec)[MCFL_SYSREADY&&MCFR_SYSREADY&&aQuitInverterOn&&bQuitInverterOn]
    MCFR_InverterOn_State -> SYSRDYCECK : after(1,sec)
    MCFL_InverterOn_State -> MCFR_InverterOn_State : after(5,sec)
    MCDCEnableState -> MCFL_InverterOn_State : after(1,sec)
  state Output [parallel]
    du:
    VehReady = in(VehStat.Ready);
    VehStandby = in(VehStat.Standby);
    BeeperStOut = in(BeeperStat.ON);
    AMKCANready = in(AMKCANenable.ON);
    MCFL_DCOn_setpoints = in(AMKDCon.ON);
    MCFR_DCOn_setpoints = in(AMKDCon.ON);
    MCFL_DCEnable = in(MCDCEnable.ON);
    MCFR_DCEnable = in(MCDCEnable.ON);
    %MC_DCOnError = in(AMKDCready.MC_DCOnFail);
    AMKMCFL_InverterOn = in(MCFL_InverterOn.ON);
    AMKMCFR_InverterOn = in(MCFR_InverterOn.ON);
    MCFL_TorqueOn = in(MC_TorqueCUT.ON);
    MCFR_TorqueOn = in(MC_TorqueCUT.ON);
    settings: executionOrder=7
  state AMKCANenable [parallel]
    settings: executionOrder=8
    state OFF
    state ON
    (default) -> AMKCANenable.OFF
    AMKCANenable.OFF -> AMKCANenable.ON : AMKCANON
    AMKCANenable.ON -> AMKCANenable.OFF : AMKCANOFF
  state MCFL_InverterOn [parallel]
    settings: executionOrder=9
    state OFF
    state ON
    (default) -> MCFL_InverterOn.OFF
    MCFL_InverterOn.OFF -> MCFL_InverterOn.ON : InverterFLON
    MCFL_InverterOn.ON -> MCFL_InverterOn.OFF : InverterFLOFF
  state MCFR_InverterOn [parallel]
    settings: executionOrder=10
    state OFF
    state ON
    (default) -> MCFR_InverterOn.OFF
    MCFR_InverterOn.OFF -> MCFR_InverterOn.ON : InverterFRON
    MCFR_InverterOn.ON -> MCFR_InverterOn.OFF : InverterFROFF
  state MC_DCOnFail [parallel] [commented out]
    en:
    send(AMKDCOFF,AMKDCon);
    send(MCDCEnableOFF,MCDCEnable);
    send(InverterOFF,MC_InverterOn);
    send(TorqueOFF,MC_TorqueCUT);
  (default) -> MC_DCOnFail [commented out] : [~MCFRDCOncheck||~MCFLDCOncheck]
  (default) -> MC_DCOnFail [commented out] : [~MCFL_SYSREADY||~MCFR_SYSREADY||~aQuitInverterOn||~bQuitInverterOn]
  data: Brk input boolean size=1; KeyPressed input boolean size=1; VehReady output boolean size=1; BeeperStOut output boolean size=1; VehStandby output boolean; ACC_Release input boolean; cMCUReady input; aMCUReady input; bMCUReady input; AMKCANready output; MCFL_DCOn_setpoints output; MCFRDCOncheck input; MCFLDCOncheck input; MCFR_DCOn_setpoints output; MCFR_DCEnable output; MCFL_DCEnable output; MCFL_SYSREADY input; MCFR_SYSREADY input; errorReset output; aQuitInverterOn input; bQuitInverterOn input; MCFR_TorqueOn output; MCFL_TorqueOn output; AMKMCFL_InverterOn output; AMKMCFR_InverterOn output
  events: EbeepON local FUNCTION_CALL_EVENT; EbeepOFF local FUNCTION_CALL_EVENT; AMKCANOFF local FUNCTION_CALL_EVENT; AMKCANON local FUNCTION_CALL_EVENT; AMKDCON local FUNCTION_CALL_EVENT; AMKDCOFF local FUNCTION_CALL_EVENT; InverterOFF local FUNCTION_CALL_EVENT; InverterON local FUNCTION_CALL_EVENT; MCDCEnableON local FUNCTION_CALL_EVENT; MCDCEnableOFF local FUNCTION_CALL_EVENT; TorqueOFF local FUNCTION_CALL_EVENT; TorqueON local FUNCTION_CALL_EVENT; InverterFROFF local FUNCTION_CALL_EVENT; InverterFLOFF local FUNCTION_CALL_EVENT; InverterFLON local FUNCTION_CALL_EVENT; InverterFRON local FUNCTION_CALL_EVENT

== matlab function VehCtrlMdel240926_2018b_amkspdlimit/CTRL/MoTrqReq/DYC/MATLAB Function ==
  data: Fz1 input; T1max output; Fz2 input; Fz3 input; Fz4 input; T2max output; T34max output; TamkFL_max input; TamkFR_max input; Temrax_max input; ay_g input; Rt input; i1 input; i2 input; u input
function [T1max,T2max,T34max] = fcn(Fz1,Fz2,Fz3,Fz4, TamkFL_max,TamkFR_max, Temrax_max,ay_g,Rt,i1,i2,u)
g = 9.8;

Fx1 = sqrt(power(Fz1*u,2)-power(Fz1*ay_g/g,2));
Fx2 = sqrt(power(Fz2*u,2)-power(Fz2*ay_g/g,2));
Fx3 = sqrt(power(Fz3*u,2)-power(Fz3*ay_g/g,2));
Fx4 = sqrt(power(Fz4*u,2)-power(Fz4*ay_g/g,2));


T1max = min(Fx2*Rt/i1,TamkFR_max);
T2max = min(Fx1*Rt/i1,TamkFL_max);
T34max = min((Fx4+Fx3)/2*Rt/i2,Temrax_max);

== stateflow chart VehCtrlMdel240926_2018b_amkspdlimit/Input_Processing/Function-Call Subsystem/AccBrkPedal/Timer ==
  state Trigger
    en:
    x = x + 0.01;
    Exit=0;
  state Out
    en:
    Exit=1;
    x=0;
  state InterState
    en:
    x=0;
  Trigger -> Trigger [order 1] : [Trigger&&x<CountTime]
  Trigger -> Out [order 2] : [x>=CountTime]
  (default) -> Trigger
  Out -> Trigger : [~Trigger]
  InterState -> Trigger : [Trigger]
  Trigger -> InterState [order 3] : [x<CountTime&&~Trigger]
  data: Trigger input; CountTime input; Exit output; x local =0

== matlab function VehCtrlMdel240926_2018b_amkspdlimit/CTRL/MoTrqReq/DYC/MATLAB Function1 ==
  data: WSA input; Mz output; WSAV input; Vx input; Iz input; Caf input; Car input; lf input; lr input; m input
function Mz = fcn(WSA,WSAV,Vx,Iz,Caf,Car,lf,lr,m)

Mz = ((((lf*lf*Caf+lr*lr*Car)/Iz/Vx)*(-Caf/m/Vx)-((lf*Caf-lr*Car)/m/Vx/Vx-1)*(-lf*Caf/Iz))*Iz*WSA-(-Caf/m/Vx)*Iz*WSAV)/((lf*Caf-lr*Car)/m/Vx/Vx-1)/100;

== stateflow chart VehCtrlMdel240926_2018b_amkspdlimit/CTRL/PwrTrainTempPrtct/Timer1 ==
  state Trigger
    en:
    x = x + 0.01;
    Exit=0;
  state Out
    en:
    Exit=1;
    x=0;
  state InterState
    en:
    x=0;
  Trigger -> Trigger [order 1] : [Trigger&&x<CountTime]
  Trigger -> Out [order 2] : [x>=CountTime]
  (default) -> Trigger
  Out -> Trigger : [~Trigger]
  InterState -> Trigger : [Trigger]
  Trigger -> InterState [order 3] : [x<CountTime&&~Trigger]
  data: Trigger input; CountTime input; Exit output; x local =0

== stateflow chart VehCtrlMdel240926_2018b_amkspdlimit/CTRL/PwrTrainTempPrtct/Timer2 ==
  state Trigger
    en:
    x = x + 0.01;
    Exit=0;
  state Out
    en:
    Exit=1;
    x=0;
  state InterState
    en:
    x=0;
  Trigger -> Trigger [order 1] : [Trigger&&x<CountTime]
  Trigger -> Out [order 2] : [x>=CountTime]
  (default) -> Trigger
  Out -> Trigger : [~Trigger]
  InterState -> Trigger : [Trigger]
  Trigger -> InterState [order 3] : [x<CountTime&&~Trigger]
  data: Trigger input; CountTime input; Exit output; x local =0

== stateflow chart VehCtrlMdel240926_2018b_amkspdlimit/CTRL/MoTrqReq/Chart ==
  state A [parallel]
    settings: executionOrder=2
    state A
      en:
      if abs(IMU_Ay)>0.5
      a=atan(IMU_Ax/IMU_Ay)*180/pi;
      else
      a = 0;
      end
      b=sqrt(power(IMU_Ax,2)+power(IMU_Ay,2));
    (default) -> A.A
    A.A -> A.A
  state B [parallel]
    settings: executionOrder=1
    state InitState
    state DYC_Disenable
      en:
      DYC_Enable_OUT=0;
      DYC_flag=0;
    state DYC_Enable
      en:
      DYC_Enable_OUT=1;
      DYC_flag=1;
    (default) -> InitState
    DYC_Disenable -> InitState : [DYC_Enable]
    InitState -> DYC_Disenable [order 2] : [~DYC_Enable]
    DYC_Enable -> InitState : [IMU_Yaw>=50||IMU_Ay>=5||b>=5]
    InitState -> DYC_Enable [order 1] : [DYC_Enable&&IMU_Yaw<=50&&IMU_Ay<5&&b<5&&IMU_Yaw_Valid&&WhlStrAng_Valid]
  state C [parallel]
    settings: executionOrder=3
    state B
      en:
      TCSR_Enable_OUT=1;
    state F_TVD_TCS_STATE
    state C
      en:
      TCSR_Enable_OUT=0;
    F_TVD_TCS_STATE -> C.B [order 1] : [DYC_flag&&IMU_Yaw<=30&&a>=30&&a<=-30&&b<=3]
    C.B -> F_TVD_TCS_STATE : [~DYC_flag||IMU_Yaw>30||a>30||a>-30||b>3]
    (default) -> F_TVD_TCS_STATE
    C.C -> F_TVD_TCS_STATE : [DYC_flag&&IMU_Yaw<=30&&a>=30&&a<=-30&&b<=3]
    F_TVD_TCS_STATE -> C.C [order 2] : [~DYC_flag||IMU_Yaw>30||a>30||a>-30||b>3]
  state D [parallel]
    settings: executionOrder=4
    state InitState2
    state TCSR_Disenable
      en:
      TCSR_Enable_OUT=0;
    state TCSR_Enable
      en:
      TCSR_Enable_OUT=1;
    (default) -> InitState2
    InitState2 -> TCSR_Disenable [order 2] : [~TCSR_Enable]
    InitState2 -> TCSR_Enable [order 1] : [TCSR_Enable]
    TCSR_Disenable -> TCSR_Enable : [TCSR_Enable]
    TCSR_Enable -> TCSR_Disenable : [~TCSR_Enable]
  state E [parallel]
    settings: executionOrder=5
    state InitState1
    state TCSF_Disenable
      en:
      TCSF_Enable_OUT=0;
    state TCSF_Enable
      en:
      TCSF_Enable_OUT=1;
    (default) -> InitState1
    TCSF_Disenable -> InitState1 : [TCSF_Enable]
    InitState1 -> TCSF_Disenable [order 2] : [~TCSF_Enable]
    InitState1 -> TCSF_Enable [order 1] : [TCSF_Enable&&DYC_flag&&~DYC_flag&&a>60&&a<-60&&IMU_Ax>2&&b<5&&IMU_Yaw<50]
    TCSF_Enable -> InitState1 : [b>5]
  data: DYC_Enable input; TCSF_Enable input; TCSR_Enable input; TCSFR_flgActv input; TCSFL_flgActv input; TCSR_flgActv input; TVD_Trigger input; DYC_Enable_OUT output; TCSR_Enable_OUT output; TCSF_Enable_OUT output; IMU_Ax input; IMU_Ay input; IMU_Yaw input; a local; b local; DYC_flag local; IMU_Yaw_Valid input; WhlStrAng_Valid input

== stateflow chart VehCtrlMdel240926_2018b_amkspdlimit/Input_Processing/Function-Call Subsystem/SWAS/Timer ==
  state Trigger
    en:
    x = x + 0.01;
    Exit=0;
  state Out
    en:
    Exit=1;
    x=0;
  state InterState
    en:
    x=0;
  Trigger -> Trigger [order 1] : [Trigger&&x<CountTime]
  Trigger -> Out [order 2] : [x>=CountTime]
  (default) -> Trigger
  Out -> Trigger : [~Trigger]
  InterState -> Trigger : [Trigger]
  Trigger -> InterState [order 3] : [x<CountTime&&~Trigger]
  data: Trigger input; CountTime input; Exit output; x local =0

== stateflow chart VehCtrlMdel240926_2018b_amkspdlimit/Input_Processing/Function-Call Subsystem/WhlSpdii_mps/Timer ==
  state Trigger
    en:
    x = x + 0.01;
    Exit=0;
  state Out
    en:
    Exit=1;
    x=0;
  state InterState
    en:
    x=0;
  Trigger -> Trigger [order 1] : [Trigger&&x<CountTime]
  Trigger -> Out [order 2] : [x>=CountTime]
  (default) -> Trigger
  Out -> Trigger : [~Trigger]
  InterState -> Trigger : [Trigger]
  Trigger -> InterState [order 3] : [x<CountTime&&~Trigger]
  data: Trigger input; CountTime input; Exit output; x local =0

== stateflow chart VehCtrlMdel240926_2018b_amkspdlimit/Input_Processing/Function-Call Subsystem/WhlSpdii_mps/Timer1 ==
  state Trigger
    en:
    x = x + 0.01;
    Exit=0;
  state Out
    en:
    Exit=1;
    x=0;
  state InterState
    en:
    x=0;
  Trigger -> Trigger [order 1] : [Trigger&&x<CountTime]
  Trigger -> Out [order 2] : [x>=CountTime]
  (default) -> Trigger
  Out -> Trigger : [~Trigger]
  InterState -> Trigger : [Trigger]
  Trigger -> InterState [order 3] : [x<CountTime&&~Trigger]
  data: Trigger input; CountTime input; Exit output; x local =0

== stateflow chart VehCtrlMdel240926_2018b_amkspdlimit/Input_Processing/Function-Call Subsystem/WhlSpdii_mps/Timer2 ==
  state Trigger
    en:
    x = x + 0.01;
    Exit=0;
  state Out
    en:
    Exit=1;
    x=0;
  state InterState
    en:
    x=0;
  Trigger -> Trigger [order 1] : [Trigger&&x<CountTime]
  Trigger -> Out [order 2] : [x>=CountTime]
  (default) -> Trigger
  Out -> Trigger : [~Trigger]
  InterState -> Trigger : [Trigger]
  Trigger -> InterState [order 3] : [x<CountTime&&~Trigger]
  data: Trigger input; CountTime input; Exit output; x local =0

== stateflow chart VehCtrlMdel240926_2018b_amkspdlimit/Input_Processing/Function-Call Subsystem/WhlSpdii_mps/Timer3 ==
  state Trigger
    en:
    x = x + 0.01;
    Exit=0;
  state Out
    en:
    Exit=1;
    x=0;
  state InterState
    en:
    x=0;
  Trigger -> Trigger [order 1] : [Trigger&&x<CountTime]
  Trigger -> Out [order 2] : [x>=CountTime]
  (default) -> Trigger
  Out -> Trigger : [~Trigger]
  InterState -> Trigger : [Trigger]
  Trigger -> InterState [order 3] : [x<CountTime&&~Trigger]
  data: Trigger input; CountTime input; Exit output; x local =0

== matlab function VehCtrlMdel240926_2018b_amkspdlimit/CTRL/MoTrqReq/DYC/Wtarget ==
  data: Vx_mps input size=1; Wtarget output size=1; WhlStrAng input size=1; btarget output; lf input; lr input; m input; Car input; Caf input; u input; Ax_mpss input
function [Wtarget,btarget] = fcn(Vx_mps,WhlStrAng,lf,lr,m,Car,Caf,u,Ax_mpss)
Wdes = Vx_mps*WhlStrAng/(lf+lr+(m*Vx_mps*Vx_mps*(lr*Car-lf*Caf)/Caf/Car/(lr+lf)/2));
Wu = 0.85*u*9.8/Ax_mpss;
temp = min(abs(Wu),abs(Wdes));
    Wtarget = temp*sign(Wdes);
%     Wtarget = Wdes;

bdes = (lr-lf*m*Vx_mps*Vx_mps/Car/(lf+lr)/2)*WhlStrAng/(lr+lf+m*Vx_mps*Vx_mps*(lr*Car-lf*Caf)/Car/Caf/(lf+lr)/2);
bu = atan(0.02*u*9.8);
if abs(bdes)<=bu
btarget = bdes;
else
    btarget = bu*sign(bdes);
end

== stateflow chart VehCtrlMdel240926_2018b_amkspdlimit/Input_Processing/Subsystem/WhlSlpageJudgment/Timer ==
  state Trigger
    en:
    x = x + 0.01;
    Exit=0;
  state Out
    en:
    Exit=1;
    x=0;
  state InterState
    en:
    x=0;
  Trigger -> Trigger [order 1] : [Trigger&&x<CountTime]
  Trigger -> Out [order 2] : [x>=CountTime]
  (default) -> Trigger
  Out -> Trigger : [~Trigger]
  InterState -> Trigger : [Trigger]
  Trigger -> InterState [order 3] : [x<CountTime&&~Trigger]
  data: Trigger input; CountTime input; Exit output; x local =0

== stateflow chart VehCtrlMdel240926_2018b_amkspdlimit/Input_Processing/Subsystem/WhlSpdSelect/Timer1 ==
  state Trigger
    en:
    x = x + 0.01;
    Exit=0;
  state Out
    en:
    Exit=1;
    x=0;
  state InterState
    en:
    x=0;
  Trigger -> Trigger [order 1] : [Trigger&&x<CountTime]
  Trigger -> Out [order 2] : [x>=CountTime]
  (default) -> Trigger
  Out -> Trigger : [~Trigger]
  InterState -> Trigger : [Trigger]
  Trigger -> InterState [order 3] : [x<CountTime&&~Trigger]
  data: Trigger input; CountTime input; Exit output; x local =0

== stateflow chart VehCtrlMdel240926_2018b_amkspdlimit/Input_Processing/Subsystem/WhlSpdSelect/Timer2 ==
  state Trigger
    en:
    x = x + 0.01;
    Exit=0;
  state Out
    en:
    Exit=1;
    x=0;
  state InterState
    en:
    x=0;
  Trigger -> Trigger [order 1] : [Trigger&&x<CountTime]
  Trigger -> Out [order 2] : [x>=CountTime]
  (default) -> Trigger
  Out -> Trigger : [~Trigger]
  InterState -> Trigger : [Trigger]
  Trigger -> InterState [order 3] : [x<CountTime&&~Trigger]
  data: Trigger input; CountTime input; Exit output; x local =0

== stateflow chart VehCtrlMdel240926_2018b_amkspdlimit/Input_Processing/Subsystem/WhlSlpageJudgment/Timer1 ==
  state Trigger
    en:
    x = x + 0.01;
    Exit=0;
  state Out
    en:
    Exit=1;
    x=0;
  state InterState
    en:
    x=0;
  Trigger -> Trigger [order 1] : [Trigger&&x<CountTime]
  Trigger -> Out [order 2] : [x>=CountTime]
  (default) -> Trigger
  Out -> Trigger : [~Trigger]
  InterState -> Trigger : [Trigger]
  Trigger -> InterState [order 3] : [x<CountTime&&~Trigger]
  data: Trigger input; CountTime input; Exit output; x local =0
